simulink model "Dummy_JH_Model"  (R2023b)
settings: Solver=VariableStepAuto  StartTime=0.0  StopTime=10.0  RelTol=1e-3
values from neighbouring files (symbols this model uses):
  D_H = [ ... (first row only)    [Dummy_URDF.m]
undefined symbols (not defined in the file or in its folder): Dummy, smiData, X, Y, Z
libraries: sm_lib x594, nesl_utility x13, robotcorelib x1, robotmaniplib x1
(part 11 of 11)

== matlab function Dummy_JH_Model/inv_kinematic/MATLAB Function5 ==
  data: T_target input; joint_thetas_ret output; joint_thetas input; D_H input
function joint_thetas_ret  = get_theta6(T_target, joint_thetas, D_H)
joint_thetas_ret = joint_thetas;
for i = 1:4
    joint_thetas_ret(i, 6) = get_theta6_(T_target, joint_thetas_ret(i, :), D_H);
end
end

function theta6_value = get_theta6_(T_target, thetas, D_H)
a_cow = D_H(:, 1);
d_cow = D_H(:, 3);
a2 = a_cow(3);
a3 = a_cow(4);
d4 = d_cow(4);
px = T_target(1,4);
py = T_target(2,4);
pz = T_target(3,4);
nx = T_target(1,1);
ny = T_target(2,1);
nz = T_target(3,1);
ox = T_target(1,2);
oy = T_target(2,2);
oz = T_target(3,2);
ax= T_target(1,3);
ay= T_target(2,3);
az= T_target(3,3);
theta2 = thetas(2);
theta3 = thetas(3);
theta1 = thetas(1);
theta4 = 0;
% deg_theta5_zyz = rad2deg(-thetas(5) + pi);
% if deg_theta5_zyz == 0 || deg_theta5_zyz == 180
%     r12 = (ox*(sin(theta1)*sin(theta4)*cos(theta2)^2*cos(theta3)^2 + sin(theta1)*sin(theta4)*cos(theta2)^2*sin(theta3)^2 + cos(theta1)*cos(theta4)*cos(theta2)*cos(theta3) + sin(theta1)*sin(theta4)*cos(theta3)^2*sin(theta2)^2 + sin(theta1)*sin(theta4)*sin(theta2)^2*sin(theta3)^2 + cos(theta1)*cos(theta4)*sin(theta2)*sin(theta3)))/(cos(theta1)^2*cos(theta2)^2*cos(theta3)^2*cos(theta4)^2 + cos(theta1)^2*cos(theta2)^2*cos(theta3)^2*sin(theta4)^2 + cos(theta1)^2*cos(theta2)^2*cos(theta4)^2*sin(theta3)^2 + cos(theta1)^2*cos(theta2)^2*sin(theta3)^2*sin(theta4)^2 + cos(theta1)^2*cos(theta3)^2*cos(theta4)^2*sin(theta2)^2 + cos(theta1)^2*cos(theta3)^2*sin(theta2)^2*sin(theta4)^2 + cos(theta1)^2*cos(theta4)^2*sin(theta2)^2*sin(theta3)^2 + cos(theta1)^2*sin(theta2)^2*sin(theta3)^2*sin(theta4)^2 + cos(theta2)^2*cos(theta3)^2*cos(theta4)^2*sin(theta1)^2 + cos(theta2)^2*cos(theta3)^2*sin(theta1)^2*sin(theta4)^2 + cos(theta2)^2*cos(theta4)^2*sin(theta1)^2*sin(theta3)^2 + cos(theta2)^2*sin(theta1)^2*sin(theta3)^2*sin(theta4)^2 + cos(theta3)^2*cos(theta4)^2*sin(theta1)^2*sin(theta2)^2 + cos(theta3)^2*sin(theta1)^2*sin(theta2)^2*sin(theta4)^2 + cos(theta4)^2*sin(theta1)^2*sin(theta2)^2*sin(theta3)^2 + sin(theta1)^2*sin(theta2)^2*sin(theta3)^2*sin(theta4)^2) - (oz*(cos(theta2)*cos(theta4)*sin(theta3) - cos(theta3)*cos(theta4)*sin(theta2)))/(cos(theta2)^2*cos(theta3)^2*cos(theta4)^2 + cos(theta2)^2*cos(theta3)^2*sin(theta4)^2 + cos(theta2)^2*cos(theta4)^2*sin(theta3)^2 + cos(theta2)^2*sin(theta3)^2*sin(theta4)^2 + cos(theta3)^2*cos(theta4)^2*sin(theta2)^2 + cos(theta3)^2*sin(theta2)^2*sin(theta4)^2 + cos(theta4)^2*sin(theta2)^2*sin(theta3)^2 + sin(theta2)^2*sin(theta3)^2*sin(theta4)^2) - (oy*(cos(theta1)*sin(theta4)*cos(theta2)^2*cos(theta3)^2 + cos(theta1)*sin(theta4)*cos(theta2)^2*sin(theta3)^2 - cos(theta4)*sin(theta1)*cos(theta2)*cos(theta3) + cos(theta1)*sin(theta4)*cos(theta3)^2*sin(theta2)^2 + cos(theta1)*sin(theta4)*sin(theta2)^2*sin(theta3)^2 - cos(theta4)*sin(theta1)*sin(theta2)*sin(theta3)))/(cos(theta1)^2*cos(theta2)^2*cos(theta3)^2*cos(theta4)^2 + cos(theta1)^2*cos(theta2)^2*cos(theta3)^2*sin(theta4)^2 + cos(theta1)^2*cos(theta2)^2*cos(theta4)^2*sin(theta3)^2 + cos(theta1)^2*cos(theta2)^2*sin(theta3)^2*sin(theta4)^2 + cos(theta1)^2*cos(theta3)^2*cos(theta4)^2*sin(theta2)^2 + cos(theta1)^2*cos(theta3)^2*sin(theta2)^2*sin(theta4)^2 + cos(theta1)^2*cos(theta4)^2*sin(theta2)^2*sin(theta3)^2 + cos(theta1)^2*sin(theta2)^2*sin(theta3)^2*sin(theta4)^2 + cos(theta2)^2*cos(theta3)^2*cos(theta4)^2*sin(theta1)^2 + cos(theta2)^2*cos(theta3)^2*sin(theta1)^2*sin(theta4)^2 + cos(theta2)^2*cos(theta4)^2*sin(theta1)^2*sin(theta3)^2 + cos(theta2)^2*sin(theta1)^2*sin(theta3)^2*sin(theta4)^2 + cos(theta3)^2*cos(theta4)^2*sin(theta1)^2*sin(theta2)^2 + cos(theta3)^2*sin(theta1)^2*sin(theta2)^2*sin(theta4)^2 + cos(theta4)^2*sin(theta1)^2*sin(theta2)^2*sin(theta3)^2 + sin(theta1)^2*sin(theta2)^2*sin(theta3)^2*sin(theta4)^2);
%     r11 = (nx*(sin(theta1)*sin(theta4)*cos(theta2)^2*cos(theta3)^2 + sin(theta1)*sin(theta4)*cos(theta2)^2*sin(theta3)^2 + cos(theta1)*cos(theta4)*cos(theta2)*cos(theta3) + sin(theta1)*sin(theta4)*cos(theta3)^2*sin(theta2)^2 + sin(theta1)*sin(theta4)*sin(theta2)^2*sin(theta3)^2 + cos(theta1)*cos(theta4)*sin(theta2)*sin(theta3)))/(cos(theta1)^2*cos(theta2)^2*cos(theta3)^2*cos(theta4)^2 + cos(theta1)^2*cos(theta2)^2*cos(theta3)^2*sin(theta4)^2 + cos(theta1)^2*cos(theta2)^2*cos(theta4)^2*sin(theta3)^2 + cos(theta1)^2*cos(theta2)^2*sin(theta3)^2*sin(theta4)^2 + cos(theta1)^2*cos(theta3)^2*cos(theta4)^2*sin(theta2)^2 + cos(theta1)^2*cos(theta3)^2*sin(theta2)^2*sin(theta4)^2 + cos(theta1)^2*cos(theta4)^2*sin(theta2)^2*sin(theta3)^2 + cos(theta1)^2*sin(theta2)^2*sin(theta3)^2*sin(theta4)^2 + cos(theta2)^2*cos(theta3)^2*cos(theta4)^2*sin(theta1)^2 + cos(theta2)^2*cos(theta3)^2*sin(theta1)^2*sin(theta4)^2 + cos(theta2)^2*cos(theta4)^2*sin(theta1)^2*sin(theta3)^2 + cos(theta2)^2*sin(theta1)^2*sin(theta3)^2*sin(theta4)^2 + cos(theta3)^2*cos(theta4)^2*sin(theta1)^2*sin(theta2)^2 + cos(theta3)^2*sin(theta1)^2*sin(theta2)^2*sin(theta4)^2 + cos(theta4)^2*sin(theta1)^2*sin(theta2)^2*sin(theta3)^2 + sin(theta1)^2*sin(theta2)^2*sin(theta3)^2*sin(theta4)^2) - (nz*(cos(theta2)*cos(theta4)*sin(theta3) - cos(theta3)*cos(theta4)*sin(theta2)))/(cos(theta2)^2*cos(theta3)^2*cos(theta4)^2 + cos(theta2)^2*cos(theta3)^2*sin(theta4)^2 + cos(theta2)^2*cos(theta4)^2*sin(theta3)^2 + cos(theta2)^2*sin(theta3)^2*sin(theta4)^2 + cos(theta3)^2*cos(theta4)^2*sin(theta2)^2 + cos(theta3)^2*sin(theta2)^2*sin(theta4)^2 + cos(theta4)^2*sin(theta2)^2*sin(theta3)^2 + sin(theta2)^2*sin(theta3)^2*sin(theta4)^2) - (ny*(cos(theta1)*sin(theta4)*cos(theta2)^2*cos(theta3)^2 + cos(theta1)*sin(theta4)*cos(theta2)^2*sin(theta3)^2 - cos(theta4)*sin(theta1)*cos(theta2)*cos(theta3) + cos(theta1)*sin(theta4)*cos(theta3)^2*sin(theta2)^2 + cos(theta1)*sin(theta4)*sin(theta2)^2*sin(theta3)^2 - cos(theta4)*sin(theta1)*sin(theta2)*sin(theta3)))/(cos(theta1)^2*cos(theta2)^2*cos(theta3)^2*cos(theta4)^2 + cos(theta1)^2*cos(theta2)^2*cos(theta3)^2*sin(theta4)^2 + cos(theta1)^2*cos(theta2)^2*cos(theta4)^2*sin(theta3)^2 + cos(theta1)^2*cos(theta2)^2*sin(theta3)^2*sin(theta4)^2 + cos(theta1)^2*cos(theta3)^2*cos(theta4)^2*sin(theta2)^2 + cos(theta1)^2*cos(theta3)^2*sin(theta2)^2*sin(theta4)^2 + cos(theta1)^2*cos(theta4)^2*sin(theta2)^2*sin(theta3)^2 + cos(theta1)^2*sin(theta2)^2*sin(theta3)^2*sin(theta4)^2 + cos(theta2)^2*cos(theta3)^2*cos(theta4)^2*sin(theta1)^2 + cos(theta2)^2*cos(theta3)^2*sin(theta1)^2*sin(theta4)^2 + cos(theta2)^2*cos(theta4)^2*sin(theta1)^2*sin(theta3)^2 + cos(theta2)^2*sin(theta1)^2*sin(theta3)^2*sin(theta4)^2 + cos(theta3)^2*cos(theta4)^2*sin(theta1)^2*sin(theta2)^2 + cos(theta3)^2*sin(theta1)^2*sin(theta2)^2*sin(theta4)^2 + cos(theta4)^2*sin(theta1)^2*sin(theta2)^2*sin(theta3)^2 + sin(theta1)^2*sin(theta2)^2*sin(theta3)^2*sin(theta4)^2);
%     theta6_value = atan2(-r12, r11);
%     theta6_value = theta6_value - pi;
%     return;
% end

r32 = - (oz*(cos(theta2)*cos(theta3) + sin(theta2)*sin(theta3)))/(cos(theta2)^2*cos(theta3)^2 + cos(theta2)^2*sin(theta3)^2 + cos(theta3)^2*sin(theta2)^2 + sin(theta2)^2*sin(theta3)^2) - (ox*(cos(theta1)*cos(theta2)*sin(theta3) - cos(theta1)*cos(theta3)*sin(theta2)))/(cos(theta1)^2*cos(theta2)^2*cos(theta3)^2 + cos(theta1)^2*cos(theta2)^2*sin(theta3)^2 + cos(theta1)^2*cos(theta3)^2*sin(theta2)^2 + cos(theta1)^2*sin(theta2)^2*sin(theta3)^2 + cos(theta2)^2*cos(theta3)^2*sin(theta1)^2 + cos(theta2)^2*sin(theta1)^2*sin(theta3)^2 + cos(theta3)^2*sin(theta1)^2*sin(theta2)^2 + sin(theta1)^2*sin(theta2)^2*sin(theta3)^2) - (oy*(cos(theta2)*sin(theta1)*sin(theta3) - cos(theta3)*sin(theta1)*sin(theta2)))/(cos(theta1)^2*cos(theta2)^2*cos(theta3)^2 + cos(theta1)^2*cos(theta2)^2*sin(theta3)^2 + cos(theta1)^2*cos(theta3)^2*sin(theta2)^2 + cos(theta1)^2*sin(theta2)^2*sin(theta3)^2 + cos(theta2)^2*cos(theta3)^2*sin(theta1)^2 + cos(theta2)^2*sin(theta1)^2*sin(theta3)^2 + cos(theta3)^2*sin(theta1)^2*sin(theta2)^2 + sin(theta1)^2*sin(theta2)^2*sin(theta3)^2);
r31 = - (nz*(cos(theta2)*cos(theta3) + sin(theta2)*sin(theta3)))/(cos(theta2)^2*cos(theta3)^2 + cos(theta2)^2*sin(theta3)^2 + cos(theta3)^2*sin(theta2)^2 + sin(theta2)^2*sin(theta3)^2) - (nx*(cos(theta1)*cos(theta2)*sin(theta3) - cos(theta1)*cos(theta3)*sin(theta2)))/(cos(theta1)^2*cos(theta2)^2*cos(theta3)^2 + cos(theta1)^2*cos(theta2)^2*sin(theta3)^2 + cos(theta1)^2*cos(theta3)^2*sin(theta2)^2 + cos(theta1)^2*sin(theta2)^2*sin(theta3)^2 + cos(theta2)^2*cos(theta3)^2*sin(theta1)^2 + cos(theta2)^2*sin(theta1)^2*sin(theta3)^2 + cos(theta3)^2*sin(theta1)^2*sin(theta2)^2 + sin(theta1)^2*sin(theta2)^2*sin(theta3)^2) - (ny*(cos(theta2)*sin(theta1)*sin(theta3) - cos(theta3)*sin(theta1)*sin(theta2)))/(cos(theta1)^2*cos(theta2)^2*cos(theta3)^2 + cos(theta1)^2*cos(theta2)^2*sin(theta3)^2 + cos(theta1)^2*cos(theta3)^2*sin(theta2)^2 + cos(theta1)^2*sin(theta2)^2*sin(theta3)^2 + cos(theta2)^2*cos(theta3)^2*sin(theta1)^2 + cos(theta2)^2*sin(theta1)^2*sin(theta3)^2 + cos(theta3)^2*sin(theta1)^2*sin(theta2)^2 + sin(theta1)^2*sin(theta2)^2*sin(theta3)^2);
theta6_value = atan2(r32, -r31);
theta6_value = theta6_value - pi;
end

== matlab function Dummy_JH_Model/inv_kinematic/MATLAB Function6 ==
  data: joint_thetas input; D_H input; theta_ret output; thetas output; theta_diffs output; best_diff_index output
function [theta_ret, thetas, theta_diffs, best_diff_index]  = get_best_joint_theta(joint_thetas, D_H)
% theta_ret: 最优一组的关节相对于初始位置的旋转角度
% thetas: 所有组的关节相对于初始位置的旋转角度
% theta_diffs：所有组的与当前关节角度变化的绝对值总和，即与当前位置的差异，其大小表示需要变化的难度
thetas = joint_thetas;
    theta_diffs = zeros(1,4);
    persistent current_theta
    if isempty(current_theta)
        current_theta = zeros(1,6);
    end

    for i = 1:4
        [theta, theta_diff] = joint_theta_change(thetas(i, :), current_theta, D_H);
        thetas(i, :) = theta;
        theta_diffs(i) = theta_diff;
    end
    [~, best_diff_index] = min(theta_diffs);
    theta_ret = thetas(best_diff_index, :);
    current_theta = theta_ret;
end

function [theta_ret, theta_diff] = joint_theta_change(theta, current_theta, D_H)
    % theta_diff: 与当前关节角度变化的绝对值总和，即与当前位置的差异，其大小表示需要变化的难度
    theta_ret = zeros(1,6);
    theta_diff = 0;
    for i = 1:6
        tmp_theta = mod(theta(i) + 360, 360);
        init_theta = mod(rad2deg(D_H(i, 4)) + 360, 360);
        theta_ret(i) = tmp_theta - init_theta;
        theta_diff = theta_diff + (7 - i) * abs(theta_ret(i) - current_theta(i)); % 与当前位置的差异
    end
end

== matlab function Dummy_JH_Model/MATLAB Function ==
  data: xyz input; T_target output; rot input
function T_target = T_target_genrate(xyz, rot)
T_target = [rot xyz; 0 0 0 1];

== matlab function Dummy_JH_Model/inv_kinematic/MATLAB Function13 ==
  data: joint_thetas input; thetas_ret output
function thetas_ret = joint_rad2deg(joint_thetas)
thetas_ret = joint_thetas;
for i = 1:4
    for j = 1:6
        thetas_ret(i,j) = rad2deg(thetas_ret(i,j));
    end
end
